simulink model "Closedloop_Control_With_Rectifier"  (Simulink 8.6)
settings: Solver=VariableStepAuto  SolverMode=SingleTasking  StartTime=0.0  StopTime=1  MaxStep=0.00001  RelTol=1e-3
undefined symbols (not defined in the file): D1, lagging, powergui, pulse, sps_lib
libraries: powerlib x10, simulink x2, powerlib_meascontrol x2
settings Model: Creator=pariz  LastModifiedBy=sajad
settings SolverCC: ZeroCrossAlgorithm=Adaptive
settings DataIOCC: LimitDataPoints=off  SaveFormat=Dataset  SignalLoggingSaveFormat=Dataset  ReturnWorkspaceOutputs=on
settings OptimizationCC: ExpressionDepthLimit=128
settings DebuggingCC: UnderspecifiedInitializationDetection=Simplified  MergeDetectMultiDrivingBlocksExec=error  MaxConsecutiveZCsMsg=none  IgnoredZcDiagnostic=none  SolverPrmCheckMsg=none  FcnCallInpInsideContextMsg=EnableAllAsError  AllowSymbolicDim=on  StateNameClashWarn=none  SFUnexpectedBacktrackingDiag=error  SFNoUnconditionalDefaultTransitionDiag=error
settings HardwareCC: ProdBitPerPointer=64  ProdLargestAtomicFloat=Float  ProdIntDivRoundTo=Zero  ProdEndianess=LittleEndian  ProdWordSize=64  ProdHWDeviceType=Intel->x86-64 (Windows64)
settings ModelReferenceCC: PropagateSignalLabelsOutOfModel=on
settings SFSimCC: SimUseLocalCustomCode=on
settings RTWCC: RTWUseLocalCustomCode=on
settings GRTTargetCC: TargetLangStandard=C99 (ISO)  CombineOutputUpdateFcns=on  GRTInterface=off
settings ConfigComp: CovMetricSettings=dwe  CovSaveCumulativeToWorkspaceVar=off  CovSaveSingleToWorkspaceVar=off  CovExternalEMLEnable=on
settings SimscapeCC: SimscapeNormalizeSystem=off

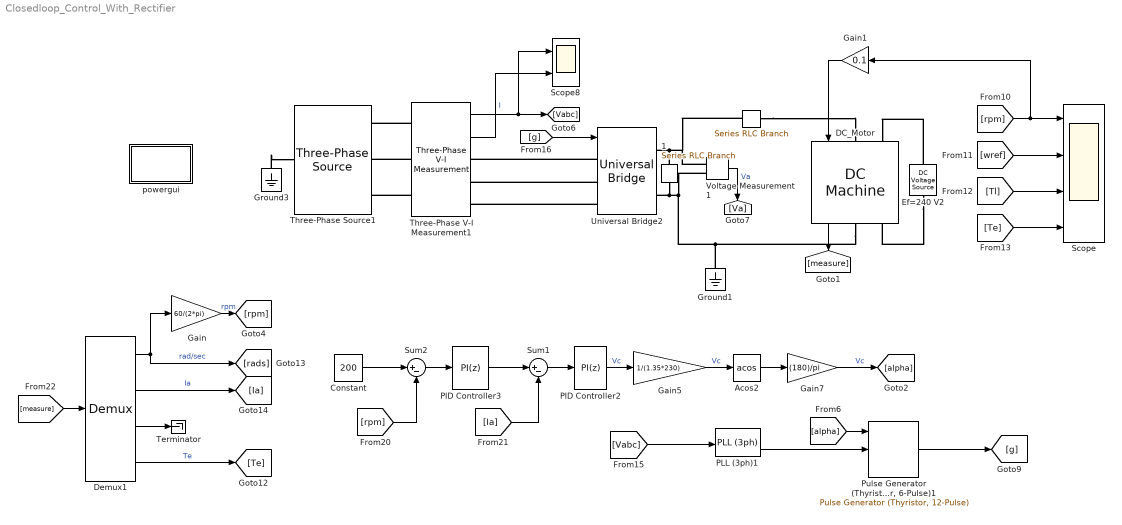
== system Closedloop_Control_With_Rectifier ==
  "   " : powerlib/Elements/Series RLC Branch  LConnTagsString=__new0  RConnTagsString=__new0  BranchType=RL  Resistance=0.001  Inductance=100e-3  SetiL0=off  InitialCurrent=0  Capacitance=1e-6  Setx0=off  InitialVoltage=0  Measurements=None
  "   1" : powerlib/Elements/Series RLC Branch  LConnTagsString=__new0  RConnTagsString=__new0  BranchType=RC  Resistance=0.001  Inductance=100e-3  SetiL0=off  InitialCurrent=0  Capacitance=800e-6  Setx0=off  InitialVoltage=0  Measurements=None
  Acos2 : Trigonometry  Operator=acos
  Constant : Constant  Value=200
  "DC_Motor " : powerlib/Machines/DC Machine  PresetModel=01: 5HP 240V 1750RPM Field:300V  MechanicalLoad=Torque TL  FieldType=Wound  ShowDetailedParameters=on  MeasurementBus=off  RLa=[2.581 0.028]  RLf=[281.2 156]  Laf=0.9483  MachineConstant=Torque constant (N.m/A)  Ke=1.8  Kt=1.8  J=0.02215  Bm=0.002953  Tf=0.5161  w0=0  Ifinit=1.06685633001422  TsPowergui=0  TsBlock=-1
      settings: AttributesFormatString=\n
  Demux1 : Demux
      settings: DisplayOption=none
  Ef=240 V2 : powerlib/Electrical Sources/DC Voltage Source  Description=source block  Amplitude=300  Measurements=None
      settings: AttributesFormatString=\n
  Gain : Gain  Gain=60/(2*pi)
  Gain1 : Gain  Gain=0.1
  Gain5 : Gain  Gain=1/(1.35*230)
  Gain7 : Gain  Gain=(180)/pi
  Ground1 : powerlib/Elements/Ground  LConnTagsString=a
  Ground3 : powerlib/Elements/Ground  LConnTagsString=a
  PID Controller2 : simulink/Continuous/PID Controller  Controller=PI  Form=Ideal  TimeDomain=Discrete-time  SampleTime=2.000000000000000e-04  IntegratorMethod=Forward Euler  ControllerParametersSource=internal  P=20  I=50  D=0  N=100  UseFilter=on  InitialConditionSource=internal  InitialConditionForIntegrator=0  InitialConditionForFilter=0  DifferentiatorICPrevScaledInput=0  ExternalReset=none  TrackingMode=off  Kt=1  LimitOutput=on  UpperSaturationLimit=300  LowerSaturationLimit=-300  LinearizeAsGain=on  AntiWindupMode=back-calculation  Kb=1  POutMin=[]  POutMax=[]  IOutMin=[]  IOutMax=[]  DOutMin=[]  DOutMax=[]  NOutMin=[]  NOutMax=[]  SumOutMin=[]  SumOutMax=[]  SaturationOutMin=[]  SaturationOutMax=[]  PParamMin=[]  PParamMax=[]  IParamMin=[]  IParamMax=[]  DParamMin=[]  DParamMax=[]  NParamMin=[]  NParamMax=[]  KbParamMin=[]  KbParamMax=[]  KtParamMin=[]  KtParamMax=[]  KbOutMin=[]  KbOutMax=[]  KtOutMin=[]  KtOutMax=[]  IntegratorOutMin=[]  IntegratorOutMax=[]  FilterOutMin=[]  FilterOutMax=[]  SumI1OutMin=[]  SumI1OutMax=[]  SumI2OutMin=[]  SumI2OutMax=[]  SumI3OutMin=[]  SumI3OutMax=[]  SumDOutMin=[]  SumDOutMax=[]  DifferentiatorOutMin=[]  DifferentiatorOutMax=[]  IntegratorContinuousStateAttributes=''  IntegratorStateMustResolveToSignalObject=off  IntegratorRTWStateStorageClass=Auto  FilterContinuousStateAttributes=''  FilterStateMustResolveToSignalObject=off  FilterRTWStateStorageClass=Auto
  PID Controller3 : simulink/Continuous/PID Controller  Controller=PI  Form=Ideal  TimeDomain=Discrete-time  SampleTime=2.000000000000000e-04  IntegratorMethod=Forward Euler  ControllerParametersSource=internal  P=0.1  I=25  D=0  N=100  UseFilter=on  InitialConditionSource=internal  InitialConditionForIntegrator=0  InitialConditionForFilter=0  DifferentiatorICPrevScaledInput=0  ExternalReset=none  TrackingMode=off  Kt=1  LimitOutput=on  UpperSaturationLimit=30  LowerSaturationLimit=0  LinearizeAsGain=on  AntiWindupMode=clamping  Kb=1  POutMin=[]  POutMax=[]  IOutMin=[]  IOutMax=[]  DOutMin=[]  DOutMax=[]  NOutMin=[]  NOutMax=[]  SumOutMin=[]  SumOutMax=[]  SaturationOutMin=[]  SaturationOutMax=[]  PParamMin=[]  PParamMax=[]  IParamMin=[]  IParamMax=[]  DParamMin=[]  DParamMax=[]  NParamMin=[]  NParamMax=[]  KbParamMin=[]  KbParamMax=[]  KtParamMin=[]  KtParamMax=[]  KbOutMin=[]  KbOutMax=[]  KtOutMin=[]  KtOutMax=[]  IntegratorOutMin=[]  IntegratorOutMax=[]  FilterOutMin=[]  FilterOutMax=[]  SumI1OutMin=[]  SumI1OutMax=[]  SumI2OutMin=[]  SumI2OutMax=[]  SumI3OutMin=[]  SumI3OutMax=[]  SumDOutMin=[]  SumDOutMax=[]  DifferentiatorOutMin=[]  DifferentiatorOutMax=[]  IntegratorContinuousStateAttributes=''  IntegratorStateMustResolveToSignalObject=off  IntegratorRTWStateStorageClass=Auto  FilterContinuousStateAttributes=''  FilterStateMustResolveToSignalObject=off  FilterRTWStateStorageClass=Auto
  PLL (3ph)1 : powerlib_meascontrol/PLL/PLL (3ph)  Fmin=45  Par_Init=[0, 60]  ParK=[180, 3200, 1]  TcD=1e-4  MaxRateChangeFreq=12  FilterCutOffFreq=25  Ts=0  AGC=on
  "Pulse Generator (Thyristor, 6-Pulse)1" : powerlib_meascontrol/Pulse & Signal Generators/Pulse Generator (Thyristor, 12-Pulse)  GenType=6-pulse  Delta=D1 (lagging)  pwidth=60  Double_Pulse=off  Ts=0
  Scope : Scope  NumInputPorts=4
  Scope8 : Scope  NumInputPorts=2
  Sum1 : Sum  Inputs=|+-
  Sum2 : Sum  Inputs=|+-
  Terminator : Terminator
  Three-Phase V-I Measurement1 : powerlib/Measurements/Three-Phase V-I Measurement  VoltageMeasurement=phase-to-ground  SetLabelV=off  LabelV=Vabc  Vpu=off  VpuLL=off  CurrentMeasurement=yes  SetLabelI=off  LabelI=Iabc  Ipu=off  Pbase=100e6  Vbase=500e3  OutputType=Complex  PhasorSimulation=off  PSBequivalent=0
  Three-Phase Source1 : powerlib/Electrical Sources/Three-Phase Source  InternalConnection=Yn  VoltagePhases=off  Voltage=230*1.73  PhaseAngle=0  Voltage_phases=[25e3 25e3 25e3]/sqrt(3)  PhaseAngles_phases=[0 -120 +120]  Frequency=60  NonIdealSource=off  SpecifyImpedance=off  Resistance=0.8929  Inductance=16.58e-3  ShortCircuitLevel=100e6  BaseVoltage=25e3  XRratio=7  BusType=swing  Pref=10e3  Qref=0  Prefabc=[10e3, 10e3, 10e3]  Qrefabc=[0, 0, 0]  Qmin=-inf  Qmax=inf
  Universal Bridge2 : powerlib/Power Electronics/Universal Bridge  Arms=3  SnubberResistance=1e5  SnubberCapacitance=inf  Device=Thyristors  Ron=1e-3  Lon=0  ForwardVoltages="[  0  0  ]"  ForwardVoltage=0  GTOparameters=[ 10e-6 , 20e-6 ]  IGBTparameters=[ 1e-6 , 2e-6 ]  Measurements=Device voltages  Measurements_2=None  converterType=Rectifier
  Voltage Measurement1 : powerlib/Measurements/Voltage Measurement  PhasorSimulation=off  OutputType=Complex  PSBequivalent=0
  powergui : Subsystem  Priority=1  AncestorBlock=sps_lib/powergui  DialogController=POWERSYS.PowerSysDialog  InitFcn=powergui( 'InitFcn_Callback' , gcb , 0 , [ ] );  mask(PSB option menu block){SimulationMode=Discrete, SampleTime=10e-6, frequency=60, Iterations=50, frequencyindice=60, Pbase=100e6, ErrMax=1e-4, UnitsV=kV, UnitsW=MW, buscounter=0, FunctionMessages=on, echomessages=on, EnableUseOfTLC=off, CurrentSourceSwitches=on, DisableSnubberDevices=on, DisableRonSwitches=on, DisableVfSwitches=on, DisplayEquations=off, AutomaticDiscreteSolvers=off, SolverType=Backward Euler, Interpol=off, ExternalGateDelay=off, methode=off, Ts=10, x0status=blocks, SPID=off, SwTol=0, HookPort=off, NonlinearTolerance=1e-4, nMaxIteration=100, ContinueOnMaxIteration=off, RestoreLinks=warning, ResistiveCurrentMeasurement=off, Frange=[0:2:500], Ylog=off, Xlog=on, ShowGrid=off, save=off, variable=ZData, structure=0, ZoomFFT=off, StartTime=0.0, cycles=1, DisplayStyle=1, fundamental=60, FreqAxis=off, MaxFrequency=1000, frequencyindicesteady=1, RmsSteady=1, display=off}
      mask prompts: SimulationMode "Simulation type:"; SampleTime "Sample time (s):"; frequency "Frequency (Hz):"; Iterations "Max iterations"; frequencyindice "Frequency (Hz)"; Pbase "Base power (VA)"; ErrMax "PQ tolerance (pu)"; UnitsV "Voltage units"; UnitsW "Power units"; buscounter "Load flow bus counter"; FunctionMessages "Disable Specialized Power Systems warnings"; echomessages "Display Specialized Power Systems compilation messages"; EnableUseOfTLC "Use TLC file when in Accelerator Simulation Mode and for code generation"; CurrentSourceSwitches "Disable ideal switching"; DisableSnubberDevices "Disable snubbers in switching devices"; DisableRonSwitches "Disable Ron resistances in switching devices"; DisableVfSwitches "Disable forward voltages in switching devices"; DisplayEquations "Display circuit differential equations"; AutomaticDiscreteSolvers "Automatically handle Discrete solver and Advanced tab solver settings of blocks"; SolverType "Discrete solver"; Interpol "Interpolate switching events"; ExternalGateDelay "Use time-stamped gate signals"; methode "Store switching topologies"; Ts "Buffer size (MBytes):"; x0status "Start simulation with initial electrical states from:"; SPID "Use ideal switching devices"; SwTol "Switch tolerance"; HookPort "Allow multiple powergui blocks"; NonlinearTolerance "Solver tolerance"; nMaxIteration "Maximum number of iterations"; ContinueOnMaxIteration "Continue Simulation if maximum number of iterations is reached"; RestoreLinks "Restore disabled links of Simscape Power Systems ST blocks:"; ResistiveCurrentMeasurement "Use non ideal current measurement blocks (1e-4Ohm internal resistance)"; Frange "Frequency Range"; Ylog "Log impedance"; Xlog "log Frequency"; ShowGrid "grid"; save "Save Data To Workspace"; variable "Variable Name"; structure "Structure Name (PSBFFTSCOPE)"; ZoomFFT "ZoomFFT (PSBFFTSCOPE)"; StartTime "Start Time (PSBFFTSCOPE)"; cycles "Cycles (PSBFFTSCOPE)"; DisplayStyle "Display style (PSBFFTSCOPE)"; fundamental "Fundamental (PSBFFTSCOPE)"; FreqAxis "Frequency Axis (PSBFFTSCOPE)"; MaxFrequency "Max Frequency (PSBFFTSCOPE)"; frequencyindicesteady "Frequency indice (STEADYSTATE)"; RmsSteady "RMS display (STEADYSTATE)"; display "Display Results"
      mask help: Set simulation type, simulation parameters, and preferences.
      mask init:
      | dispMessage = powergui('MaskInitialization',gcb,SimulationMode,SampleTime);
      settings: PreSaveFcn=powergui( 'PreSaveFcn_Callback' , gcb , [ ] , [ ] );  OpenFcn=sps_rtmsupport('OpenFcn',gcbh)
      mask Help: helpview(psbhelp)
      mask TypeOptions SimulationMode: Continuous | Discrete | Phasor | Discrete phasor
      mask Callback SimulationMode: powergui('SimulationType',[],[],gcb);
      mask TypeOptions UnitsV: V | kV
      mask TypeOptions UnitsW: W | kW | MW
      mask Callback CurrentSourceSwitches: powergui('SimulationType',[],[],gcb);
      mask Callback AutomaticDiscreteSolvers: powergui('SimulationType',[],[],gcb);
      mask TypeOptions SolverType: Tustin/Backward Euler (TBE) | Tustin | Backward Euler
      mask Callback SolverType: powergui('SimulationType',[],[],gcb);
      mask Callback Interpol: powergui('SimulationType',[],[],gcb);
      mask Callback ExternalGateDelay: powergui('SimulationType',[],[],gcb);
      mask Callback methode: powergui('SimulationType',[],[],gcb);
      mask TypeOptions x0status: blocks | steady | zero
      mask TypeOptions RestoreLinks: yes | warning | no
      mask Callback display: sps_rtmsupport('parametereditingmodes',gcbh) % Will be executed last in parameter callbacks to ensure mask enable consistency
      mask DialogControl AutoSolverNote Prompt: The Simulation type parameter is governed by Simulink. To access the Powergui solver settings, unselect auto (Automatic solver selection) solver in the Simulink solver options.
      mask DialogControl StateAnalyzer Prompt: Measurements and States Analyzer
      mask DialogControl StateAnalyzer Callback: powerStates(bdroot(gcb))
      mask DialogControl RLCLineParameters Prompt: Power Line Parameters
      mask DialogControl RLCLineParameters Callback:
      | close_system(gcb)
      | powerLineParameters
      mask DialogControl Control15 Prompt: Power Cable Parameters
      mask DialogControl Control15 Callback:
      | close_system(gcb)
      | powerCableParameters
      mask DialogControl DecouplingLines Prompt: Specify Decoupling Lines
      mask DialogControl DecouplingLines Tooltip: Click to replace selected Distributed Parameters Line blocks with Decoupling Line blocks
      mask DialogControl DecouplingLines Callback:
      | close_system(gcb);
      | DecouplingLineReplace(gcs)
      mask DialogControl LoadFlow Prompt: Load Flow Analyzer
      mask DialogControl LoadFlow Callback:
      | close_system(gcb)
      | powerLoadFlow
      mask DialogControl Container11 Prompt: Load Flow Parameters
      mask DialogControl MachineInitialization Prompt: Machine Initialization
      mask DialogControl MachineInitialization Callback:
      | close_system(gcb)
      | powericon('machineInitTool',bdroot(gcb),gcb)
      mask DialogControl ImpedanceMeasurement Prompt: Impedance Measurement
      mask DialogControl ImpedanceMeasurement Callback:
      | close_system(gcb);
      | powerImpedance(bdroot(gcs));
      mask DialogControl FFTAnalysis Prompt: FFT Analysis
      mask DialogControl FFTAnalysis Callback:
      | close_system(gcb)
      | power_fftscope(bdroot(gcb),gcb)
      mask DialogControl LinearSystemAnalyzer Prompt: Use Linear System Analyzer
      mask DialogControl LinearSystemAnalyzer Callback:
      | close_system(gcb)
      | power_ltiview(bdroot(gcb))
      mask DialogControl HysteresisDesign Prompt: Hysteresis Design
      mask DialogControl HysteresisDesign Callback:
      | close_system(gcb)
      | powerHysteresis('hysteresis.mat')
      mask DialogControl Control14 Prompt: Customize SPS blocks
      mask DialogControl Control14 Callback:
      | close_system(gcb);
      | power_customize;
      mask DialogControl GenerateReprot Prompt: Generate Report
      mask DialogControl GenerateReprot Callback:
      | close_system(gcb)
      | power_report(bdroot(gcb))
      mask DialogControl Solver Prompt: Solver
      mask DialogControl SolverDetails Prompt: Solver details for nonlinear elements
      mask Display: color('blue'),disp(dispMessage)
  wires:
  Gain1/1 -> "DC_Motor "/1
  [g] -> Universal Bridge2/1
  Three-Phase V-I Measurement1/1 -> Scope8/1, [Vabc]
  Three-Phase V-I Measurement1/2 -> Scope8/2  "I"
  Voltage Measurement1/1 -> [Va]  "Va"
  [Vabc] -> PLL (3ph)1/1
  PLL (3ph)1/2 -> "Pulse Generator (Thyristor, 6-Pulse)1"/2
  [alpha] -> "Pulse Generator (Thyristor, 6-Pulse)1"/1
  "Pulse Generator (Thyristor, 6-Pulse)1"/1 -> [g]
  [measure] -> Demux1/1
  Gain5/1 -> Acos2/1  "Vc"
  Demux1/1 -> [rads], Gain/1  "rad/sec"
  [wref] -> Scope/2
  Sum1/1 -> PID Controller2/1
  Gain/1 -> [rpm]  "rpm"
  Sum2/1 -> PID Controller3/1
  [Te] -> Scope/4
  [rpm] -> Sum2/2
  [Tl] -> Scope/3
  [rpm] -> Gain1/1, Scope/1
  [Ia] -> Sum1/2
  PID Controller3/1 -> Sum1/1
  Demux1/3 -> Terminator/1
  PID Controller2/1 -> Gain5/1  "Vc"
  Acos2/1 -> Gain7/1
  Constant/1 -> Sum2/1
  Demux1/4 -> [Te]  "Te"
  Demux1/2 -> [Ia]  "Ia"
  Gain7/1 -> [alpha]  "Vc"
  "DC_Motor "/1 -> [measure]
  connections:
  Ground1/LConn1 -- "DC_Motor "/RConn1 -- Voltage Measurement1/LConn2 -- "   1"/RConn1 -- Universal Bridge2/RConn2
  Universal Bridge2/RConn1 -- "   "/LConn1 -- Voltage Measurement1/LConn1 -- "   1"/LConn1
  Universal Bridge2/LConn2 -- Three-Phase V-I Measurement1/RConn2
  Three-Phase V-I Measurement1/LConn2 -- Three-Phase Source1/RConn2
  Universal Bridge2/LConn3 -- Three-Phase V-I Measurement1/RConn3
  "   "/RConn1 -- "DC_Motor "/LConn1
  Ef=240 V2/RConn1 -- "DC_Motor "/LConn2
  Three-Phase V-I Measurement1/LConn1 -- Three-Phase Source1/RConn1
  Universal Bridge2/LConn1 -- Three-Phase V-I Measurement1/RConn1
  Ef=240 V2/LConn1 -- "DC_Motor "/RConn2
  Ground3/LConn1 -- Three-Phase Source1/LConn1
  Three-Phase V-I Measurement1/LConn3 -- Three-Phase Source1/RConn3

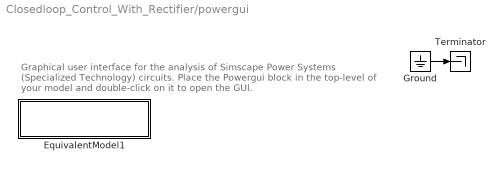
== system Closedloop_Control_With_Rectifier/powergui ==
  note: Graphical user interface for the analysis of
      | Simscape Power Systems (Specialized Technology) circuits.
      | Place the Powergui block in the top-level of your model and double-click
      | on it to open the GUI.
  EquivalentModel1 : Subsystem
      mask init:
      | S  = GetDataForEquivalentModel('Discrete',gcbh);
      mask Display:
      | color('red')
      | disp('EQUIVALENT CIRCUIT\nDiscrete')
  Ground : Ground
  Terminator : Terminator
  wires:
  Ground/1 -> Terminator/1

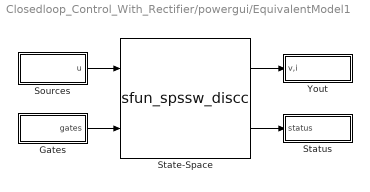
== system Closedloop_Control_With_Rectifier/powergui/EquivalentModel1 ==
  Gates : Subsystem
  Sources : Subsystem
  State-Space : S-Function  FunctionName=sfun_spssw_discc  Parameters=S.Ts,S.A, S.B, S.C, S.D, S.x0, S.EnableUseOfTLC,S.SwitchResistance ,S.SwitchType, S.SwitchGateInitialValue, S.OutputsToResetToZero, S.TBEON,S.SaveMatrices,S.BufferSize  SFunctionDeploymentMode=off  EnableBusSupport=off
  Status : Subsystem
  Yout : Subsystem
  wires:
  Gates/1(gates) -> State-Space/2
  Sources/1(u) -> State-Space/1
  State-Space/2 -> Status/1(status)
  State-Space/1 -> Yout/1(v,i)

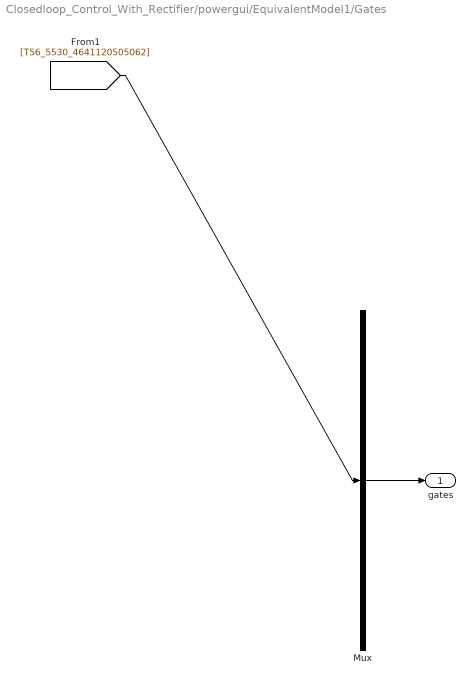
== system Closedloop_Control_With_Rectifier/powergui/EquivalentModel1/Gates ==
  Mux : Mux  Inputs=1
  gates : Outport
  wires:
  Mux/1 -> gates/1
  [T56_5530_4641120505062] -> Mux/1

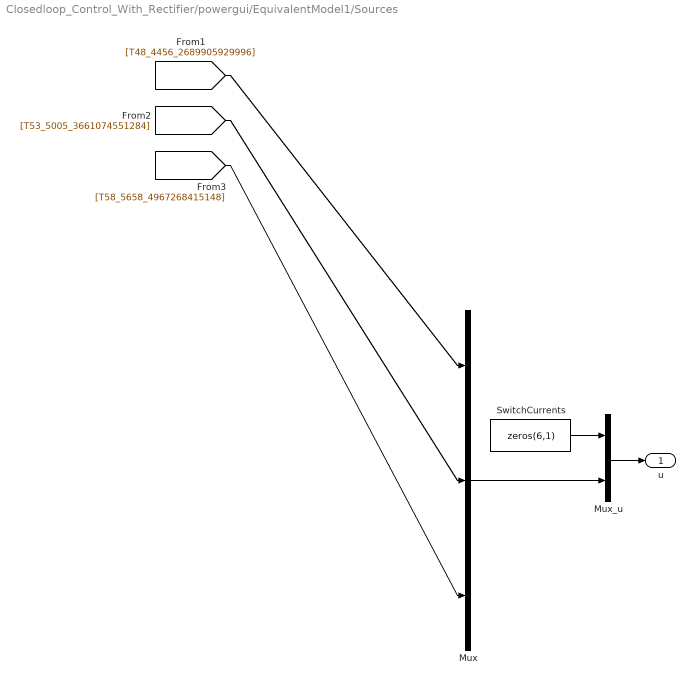
== system Closedloop_Control_With_Rectifier/powergui/EquivalentModel1/Sources ==
  Mux : Mux  Inputs=[1 1 3]
  Mux_u : Mux  Inputs=[6 5]
  SwitchCurrents : Constant  Value=zeros(6,1)
  u : Outport
  wires:
  Mux_u/1 -> u/1
  SwitchCurrents/1 -> Mux_u/1
  Mux/1 -> Mux_u/2
  [T48_4456_2689905929996] -> Mux/1
  [T53_5005_3661074551284] -> Mux/2
  [T58_5658_4967268415148] -> Mux/3

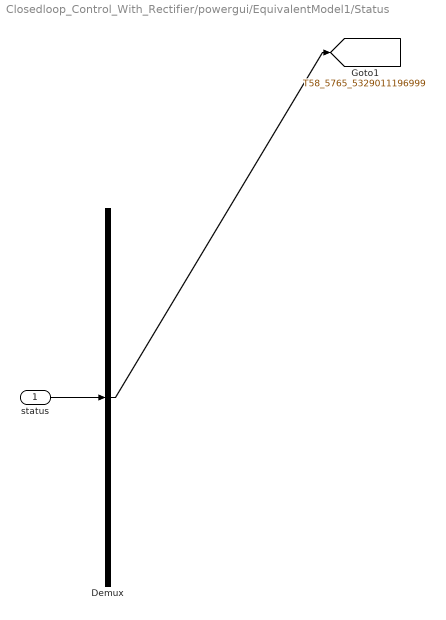
== system Closedloop_Control_With_Rectifier/powergui/EquivalentModel1/Status ==
  status : Inport
  Demux : Demux  Outputs=1
  tag scope: T58_5765_5329011196999=global
  wires:
  status/1 -> Demux/1
  Demux/1 -> [T58_5765_5329011196999]

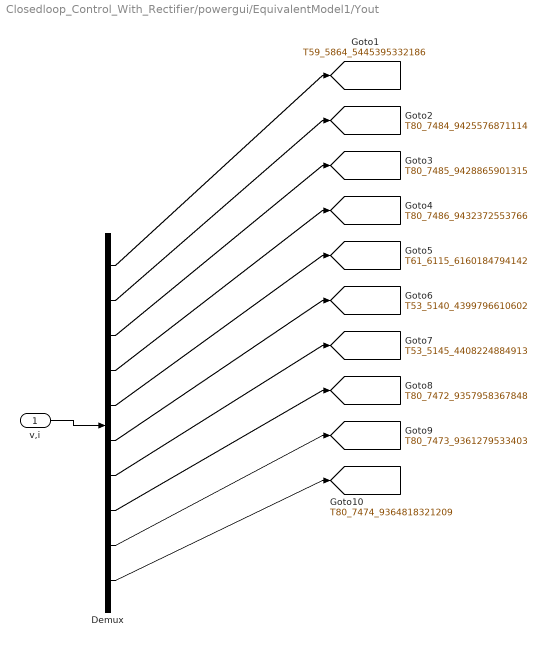
== system Closedloop_Control_With_Rectifier/powergui/EquivalentModel1/Yout ==
  v,i : Inport
  Demux : Demux  Outputs=[6 1 1 1 1 1 1 1 1 1]
  tag scope: T53_5140_4399796610602=global, T53_5145_4408224884913=global, T59_5864_5445395332186=global, T61_6115_6160184794142=global, T80_7472_9357958367848=global, T80_7473_9361279533403=global, T80_7474_9364818321209=global, T80_7484_9425576871114=global, T80_7485_9428865901315=global, T80_7486_9432372553766=global
  wires:
  v,i/1 -> Demux/1
  Demux/1 -> [T59_5864_5445395332186]
  Demux/2 -> [T80_7484_9425576871114]
  Demux/3 -> [T80_7485_9428865901315]
  Demux/4 -> [T80_7486_9432372553766]
  Demux/5 -> [T61_6115_6160184794142]
  Demux/6 -> [T53_5140_4399796610602]
  Demux/7 -> [T53_5145_4408224884913]
  Demux/8 -> [T80_7472_9357958367848]
  Demux/9 -> [T80_7473_9361279533403]
  Demux/10 -> [T80_7474_9364818321209]
